simulink model "example_udp"  (R2015a)
settings: Solver=ode4  StartTime=0.0  StopTime=inf  FixedStep=0.01  RelTol=1e-3
libraries: xpcrtudplib x1, dspnetwork x1
settings Model: Creator=ttcl3  LastModifiedBy=David
settings DataIOCC: SignalLoggingSaveFormat=ModelDataLogs
settings OptimizationCC: ExpressionDepthLimit=2147483647
settings DebuggingCC: UnderspecifiedInitializationDetection=Classic  MergeDetectMultiDrivingBlocksExec=none  SolverPrmCheckMsg=warning  FcnCallInpInsideContextMsg=UseLocalSettings  StateNameClashWarn=warning
settings GRTTargetCC: CombineOutputUpdateFcns=off  GRTInterface=on

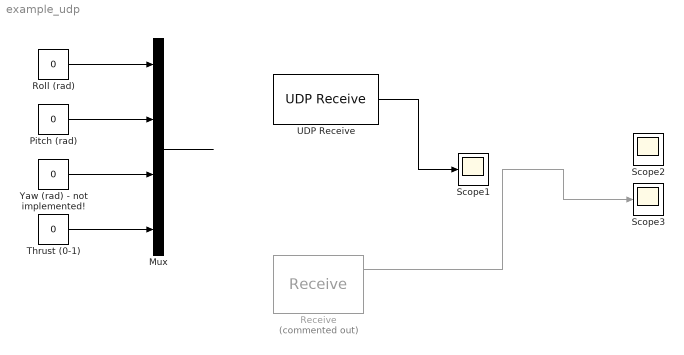
== system example_udp ==
  Mux : Mux
  Pitch (rad) : Constant  Value=0
  "Receive " : xpcrtudplib/Legacy UDP/Receive   Commented=on  ipAddress=127.0.0.1  ipPort=49000  width=100  vblLen=off  sampletime=0.01
  Roll (rad) : Constant  Value=0
  Scope1 : Scope
      settings: YMin=-0.1  YMax=0.1
  Scope2 : Scope
      settings: YMin=-0.85  YMax=0.15
  Scope3 : Scope
      settings: YMin=-0.85  YMax=0.15  SaveName=ScopeData3
  Thrust (0-1) : Constant  Value=0
  UDP Receive : dspnetwork/UDP Receive  localURL='0.0.0.0'  localPort=49000  remoteURL='127.0.0.1'  remotePort=-1  recvBufferSize=8192  dims=255  signalDatatype=single  isVarSize=on  showBlockingTime=off  blockingTime=0  sampletime=1
  Yaw (rad) - not implemented! : Constant  Value=0
  wires:
  Mux/1 -> ?
  Roll (rad)/1 -> Mux/1
  Pitch (rad)/1 -> Mux/2
  Yaw (rad) - not implemented!/1 -> Mux/3
  Thrust (0-1)/1 -> Mux/4
  ? -> Scope2/1
  "Receive "/1 -> Scope3/1
  UDP Receive/1 -> Scope1/1
